simulink model "pole_placement_1dof"  (R2023b)
settings: Solver=FixedStepAuto  StartTime=0.0  StopTime=Tend_slk  RelTol=1e-3
values from neighbouring files (symbols this model uses):
  Kv = K(:,3)    [quadcopterMain_1dof.m]
  Kx = K(:,1:2)    [quadcopterMain_1dof.m]
  L = double(L)    [H2_control_1dof.m]    (also in quadcopterMain_1dof.m = place(linsys.A',linsys.C',[-50.7 -50.6])')
  linsys = linearize(mdl,blockpath)    [quadcopterMain_1dof.m]
  param = [Ixx;Iyy;Izz;l;k;b;m]    [quadcopterMain_1dof.m]
  Ts_slk = 0.01    [quadcopterMain_1dof.m]
  x0 = [0;0]    [quadcopterMain_1dof.m]
settings Model: Creator=asus  LastModifiedBy=asus
settings OptimizationCC: ReuseModelBlockBuffer=off

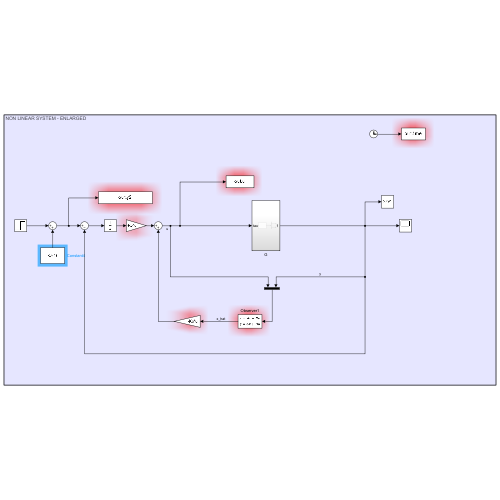
[thumbnail: Simulink's stored preview of the top-level diagram]
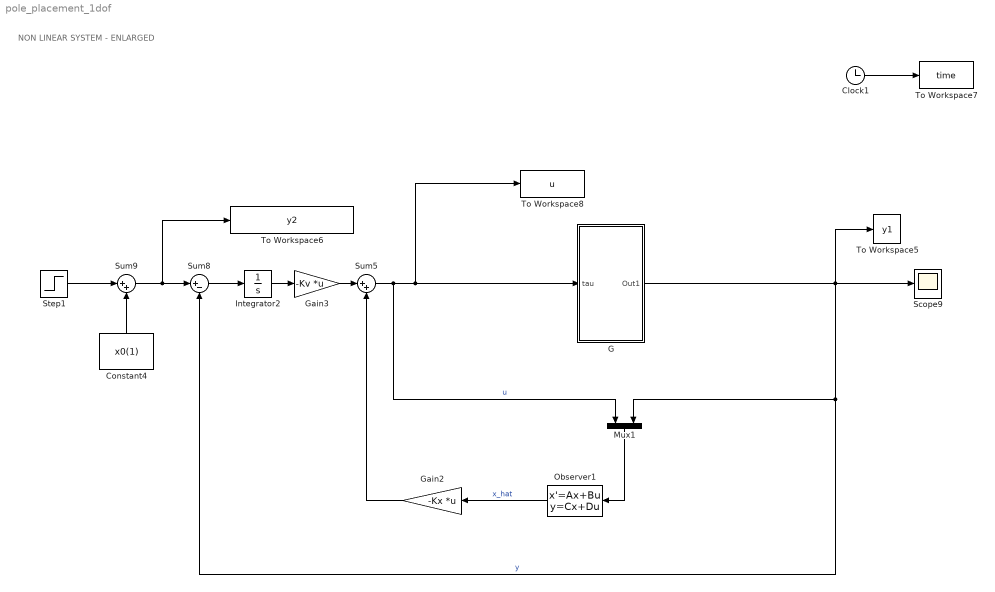
== system pole_placement_1dof ==
  note: NON LINEAR SYSTEM - ENLARGED
  Clock1 : Clock
  Constant4 : Constant  Value=x0(1)
  G : Subsystem
  Gain2 : Gain  Gain=-Kx  Multiplication=Matrix(K*u)
  Gain3 : Gain  Gain=-Kv  Multiplication=Matrix(K*u)
  Integrator2 : Integrator
  Mux1 : Mux  Inputs=2
  Observer1 : StateSpace  A=linsys.A-L*linsys.C  B=[linsys.B-L*linsys.D L]  C=eye(2)  D=zeros(2,2)  InitialCondition=0
  Scope9 : Scope
  Step1 : Step  After=30*pi/180  SampleTime=0
  Sum5 : Sum  Inputs=|++
  Sum8 : Sum  Inputs=|+-
  Sum9 : Sum  Inputs=|++
  To Workspace5 : ToWorkspace  VariableName=y1  SampleTime=-1
      settings: Save2DSignal=2-D array (concatenate along first dimension)
  To Workspace6 : ToWorkspace  VariableName=y2  SampleTime=Ts_slk
  To Workspace7 : ToWorkspace  VariableName=time  SampleTime=Ts_slk
      settings: Save2DSignal=2-D array (concatenate along first dimension)
  To Workspace8 : ToWorkspace  VariableName=u  SampleTime=Ts_slk
  wires:
  G/1(Out1) -> Mux1/2, Sum8/2, Scope9/1, To Workspace5/1  "y"
  Observer1/1 -> Gain2/1  "x_hat"
  Mux1/1 -> Observer1/1
  Sum8/1 -> Integrator2/1
  Gain2/1 -> Sum5/2
  Gain3/1 -> Sum5/1
  Sum9/1 -> To Workspace6/1, Sum8/1
  Sum5/1 -> Mux1/1, G/1("tau "), To Workspace8/1  "u"
  Constant4/1 -> Sum9/2
  Clock1/1 -> To Workspace7/1
  Integrator2/1 -> Gain3/1
  Step1/1 -> Sum9/1

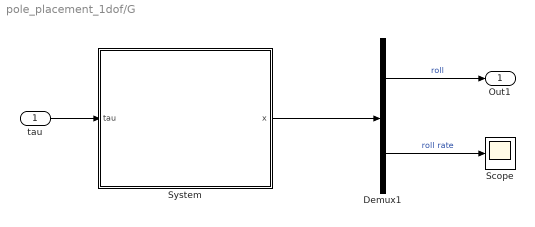
== system pole_placement_1dof/G ==
  "tau " : Inport
  Demux1 : Demux  Outputs=2
  Scope : Scope
  System : Subsystem
  Out1 : Outport
  wires:
  Demux1/1 -> Out1/1  "roll"
  "tau "/1 -> System/1("tau ")
  System/1(x) -> Demux1/1
  Demux1/2 -> Scope/1  "roll rate"

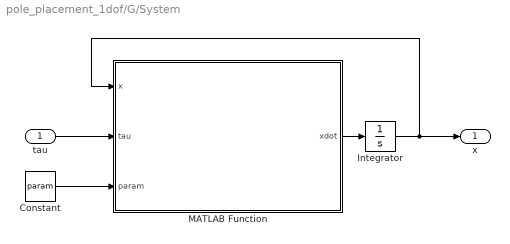
== system pole_placement_1dof/G/System ==
  "tau " : Inport
  Constant : Constant  Value=param
  Integrator : Integrator  InitialCondition=x0
  MATLAB Function : MATLAB Function  TreatAsAtomicUnit=on
  x : Outport
  wires:
  Integrator/1 -> MATLAB Function/1(x), x/1
  MATLAB Function/1(xdot) -> Integrator/1
  "tau "/1 -> MATLAB Function/2(tau)
  Constant/1 -> MATLAB Function/3(param)

== matlab function pole_placement_1dof/G/System/MATLAB Function ==
  data: x input; tau input; xdot output; param input
function xdot=quadcopter(x,tau,param)
% Inputs:
%           x       (model state)
%           tau     (torque)           
%           param   (model parameters)
%
% Outputs:  x_dot  (derivative of the state with respect to time)

% Parameters
g        =       9.81;           %  gravity acceleration (m/s^2)
Ixx      =       param(1,1);     %  moment of inertia 

% States
phi         =       x(1,1);      %  roll angle (rad)
phi_dot     =       x(2,1);      %  roll rate (rad/s)


cph         =       cos(phi);
sph         =       sin(phi);

% State space model
xdot        = zeros(2,1);
xdot(1,1)   = phi_dot;
xdot(2,1)   = tau/Ixx;
